simulink model "P_Batista"  (R2019a)
settings: Solver=VariableStepAuto  StartTime=0.0  StopTime=30  RelTol=1e-3
values from neighbouring files (symbols this model uses):
  Kalman_OP = Setup_Kalman_OP(Q, R)    [Replay_Script.m]
  sampleTime = 0.05    [Replay_Script.m]    (also in Validations_Script.m)
libraries: simulink x2
settings Model: Creator=Gaming  LastModifiedBy=Gaming

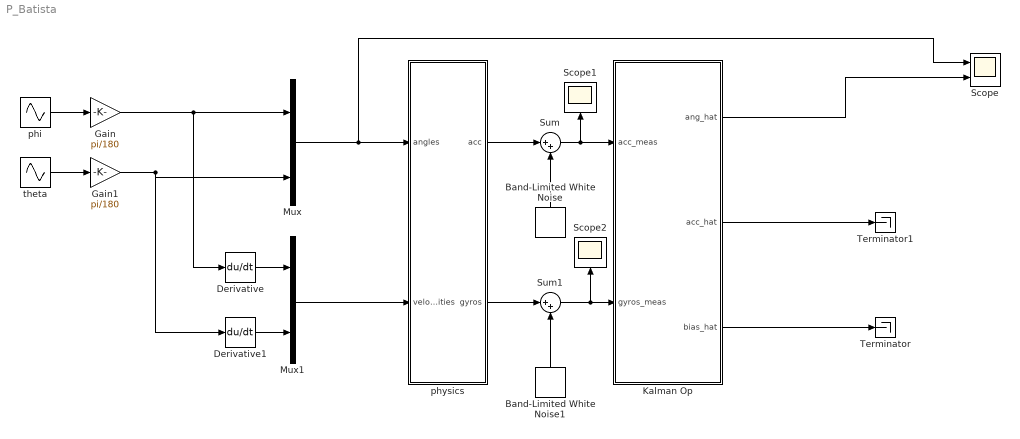
== system P_Batista ==
  Band-Limited White Noise : simulink/Sources/Band-Limited White Noise  Cov=[0.05^2*sampleTime]  Ts=sampleTime  seed=[23331]
  Band-Limited White Noise1 : simulink/Sources/Band-Limited White Noise  Cov=[(0.05*pi/180)^2*sampleTime]  Ts=sampleTime  seed=[23341]
  Derivative : Derivative
  Derivative1 : Derivative
  Gain : Gain  Gain=pi/180
  Gain1 : Gain  Gain=pi/180
  Kalman Op : Subsystem
  Mux : Mux  Inputs=2
  Mux1 : Mux  Inputs=2
  Scope : Scope  NumInputPorts=2
  Scope1 : Scope
  Scope2 : Scope
  Sum : Sum  Inputs=|++
  Sum1 : Sum  Inputs=|++
  Terminator : Terminator
  Terminator1 : Terminator
  phi : Sin  Amplitude=12  Bias=6  SampleTime=0
  physics : MATLAB Function  TreatAsAtomicUnit=on
  theta : Sin  Amplitude=25  SampleTime=0
  wires:
  phi/1 -> Gain/1
  theta/1 -> Gain1/1
  Gain/1 -> Derivative/1, Mux/1
  Gain1/1 -> Derivative1/1, Mux/2
  Mux/1 -> Scope/1, physics/1(angles)
  Mux1/1 -> physics/2(velocities)
  Derivative/1 -> Mux1/1
  Derivative1/1 -> Mux1/2
  physics/1(acc) -> Sum/1
  physics/2(gyros) -> Sum1/1
  Kalman Op/3(bias_hat) -> Terminator/1
  Kalman Op/2(acc_hat) -> Terminator1/1
  Kalman Op/1(ang_hat) -> Scope/2
  Sum/1 -> Scope1/1, Kalman Op/1(acc_meas)
  Sum1/1 -> Scope2/1, Kalman Op/2(gyros_meas)
  Band-Limited White Noise/1 -> Sum/2
  Band-Limited White Noise1/1 -> Sum1/2

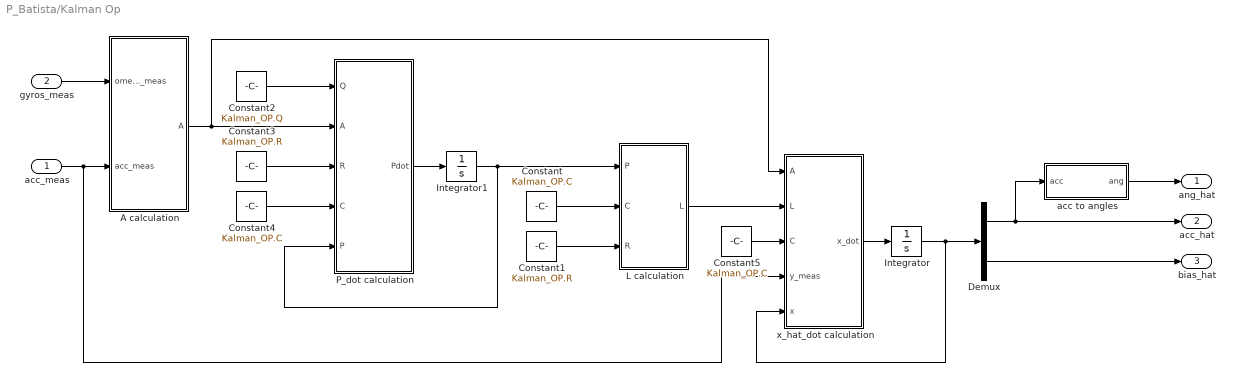
== system P_Batista/Kalman Op ==
  acc_meas : Inport
  gyros_meas : Inport  Port=2
  A calculation : MATLAB Function  TreatAsAtomicUnit=on
  Constant : Constant  Value=Kalman_OP.C
  Constant1 : Constant  Value=Kalman_OP.R
  Constant2 : Constant  Value=Kalman_OP.Q
  Constant3 : Constant  Value=Kalman_OP.R
  Constant4 : Constant  Value=Kalman_OP.C
  Constant5 : Constant  Value=Kalman_OP.C
  Demux : Demux  Outputs=2
  Integrator : Integrator  InitialCondition=zeros(6,1)
  Integrator1 : Integrator  InitialCondition=Kalman_OP.Q*10
  L calculation : MATLAB Function  TreatAsAtomicUnit=on
  P_dot calculation : MATLAB Function  TreatAsAtomicUnit=on
  acc to angles : MATLAB Function  TreatAsAtomicUnit=on
  x_hat_dot calculation : MATLAB Function  TreatAsAtomicUnit=on
  ang_hat : Outport
  acc_hat : Outport  Port=2
  bias_hat : Outport  Port=3
  wires:
  acc to angles/1(ang) -> ang_hat/1
  x_hat_dot calculation/1(x_dot) -> Integrator/1
  Integrator/1 -> Demux/1, x_hat_dot calculation/5(x)
  L calculation/1(L) -> x_hat_dot calculation/2(L)
  P_dot calculation/1(Pdot) -> Integrator1/1
  Integrator1/1 -> P_dot calculation/5(P), L calculation/1(P)
  Constant/1 -> L calculation/2(C)
  Constant1/1 -> L calculation/3(R)
  Constant3/1 -> P_dot calculation/3(R)
  Constant2/1 -> P_dot calculation/1(Q)
  Demux/1 -> acc to angles/1(acc), acc_hat/1
  Demux/2 -> bias_hat/1
  acc_meas/1 -> x_hat_dot calculation/4(y_meas), A calculation/2(acc_meas)
  gyros_meas/1 -> A calculation/1(omega_meas)
  A calculation/1(A) -> x_hat_dot calculation/1(A), P_dot calculation/2(A)
  Constant4/1 -> P_dot calculation/4(C)
  Constant5/1 -> x_hat_dot calculation/3(C)

== matlab function P_Batista/Kalman Op/P_dot calculation ==
  data: Q input; A input; Pdot output; R input; C input; P input
function Pdot = fcn(Q, A, R, C, P)

Pdot = A*P + P*A + Q - P*transpose(C)*inv(R)*C*P;

== matlab function P_Batista/physics ==
  data: angles input; acc output; velocities input; gyros output
function [acc,gyros] = fcn(angles, velocities)

% angles - phi, theta

acc = -10*[-sin(angles(2)); cos(angles(2))*sin(angles(1));cos(angles(2))*cos(angles(1))];

A = [1, sin(velocities(1))*tan(velocities(2))   , cos(velocities(1))*tan(velocities(2)) ;...
     0, cos(velocities(1))                      , -sin(velocities(1))                   ;...
     0, sin(velocities(1))/cos(velocities(2))   , cos(velocities(1))/cos(velocities(2))];


gyros = A\[velocities;0];

== matlab function P_Batista/Kalman Op/acc to angles ==
  data: acc input; ang output
function ang = fcn(acc)

phi = -atan2(acc(2),-acc(3));

theta = atan2(acc(1),sqrt(acc(2)^2+acc(3)^2));

ang = [phi; theta];

== matlab function P_Batista/Kalman Op/L calculation ==
  data: P input; L output; C input; R input
function L = fcn(P, C, R)

L = P*transpose(C)*inv(R);

== matlab function P_Batista/Kalman Op/x_hat_dot calculation ==
  data: A input; x_dot output; L input; C input; y_meas input; x input
function x_dot = fcn(A,L,C,y_meas,x)

x_dot = A*x + L*(y_meas - C*x);

== matlab function P_Batista/Kalman Op/A calculation ==
  data: omega_meas input; A output; acc_meas input
function A = fcn(omega_meas, acc_meas)

w = omega_meas;
a = acc_meas;

s_1 = [ 0   , -w(3) ,  w(2) ;...
        w(3),  0    , -w(1) ;...
       -w(2),  w(1) ,  0    ];
   
s_2 = [ 0   , -a(3) ,  a(2) ;...
        a(3),  0    , -a(1) ;...
       -a(2),  a(1) ,  0    ];
   
A = [-s_1, -s_2 ;...
     zeros(3,6) ];
